simulink model "UAV_6DOF"  (R2024b)
settings: Solver=ode3  StartTime=0.0  StopTime=5.0  FixedStep=0.001  RelTol=1e-3
model workspace (MAT data in the model file):
  Kd_roll = 0.2
  Kd_x = 2
  Kd_y = 1
  Kd_z = 0.3
  Kp_pitch = 0.5
  Kp_roll = 0.5
  Kp_x = 0.9
  Kp_y = -0.9
  Kp_z = -0.9
values from neighbouring files (symbols this model uses):
  mass = 1.5 + rand*0.5    [MonteCarlo.m]
libraries: shared6dof x1
settings Model: Creator=nikhilranjit  LastModifiedBy=nikhilranjit

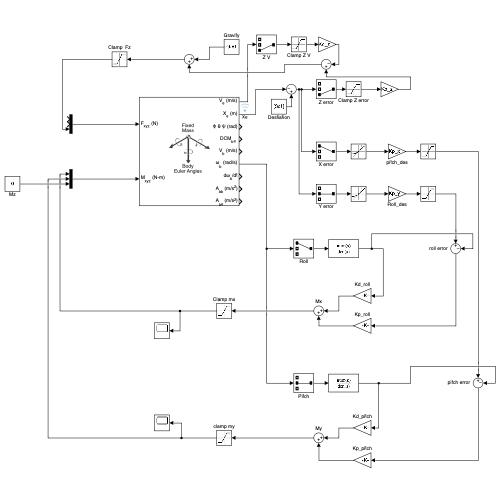
[thumbnail: Simulink's stored preview of the top-level diagram]
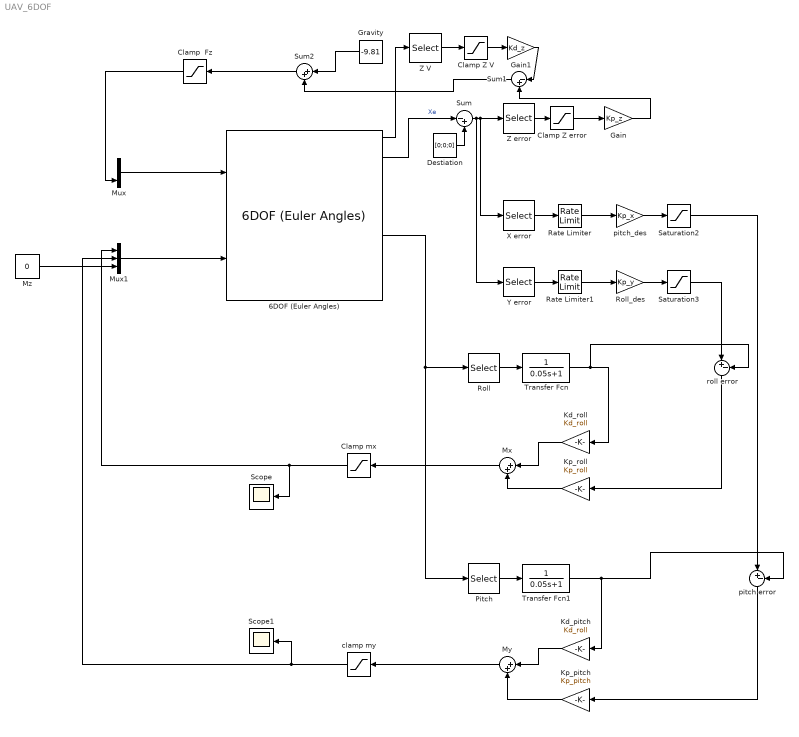
== system UAV_6DOF ==
  6DOF (Euler Angles) : shared6dof/6DOF (Euler Angles)  units=Metric (MKS)  mtype=Fixed  rep=Euler Angles  xme_0=[10 10 0]  Vm_0=[0 0 0]  eul_0=[0 0 0]  pm_0=[0 0 0]  mass_0=1.0  mass_e=0.5  mass_f=2.0  inertia=eye(3)  inertia_e=eye(3)  inertia_f=2*eye(3)  k_quat=1.0  vre_flag=on  abi_flag=on  aMode=0  xme_statename=''  Vm_statename=''  eul_statename=''  quat_statename=''  pm_statename=''  mass_statename=''
  Clamp  Fz : Saturate  UpperLimit=mass*9.81*1.5  LowerLimit=mass*9.81*0.8
  Clamp Z V : Saturate  UpperLimit=5  LowerLimit=-5
  Clamp Z error : Saturate  UpperLimit=5  LowerLimit=-5
  Clamp mx : Saturate  UpperLimit=5  LowerLimit=-5
  Destiation : Constant  Value=[0;0;0]
  Gain : Gain  Gain=Kp_z
  Gain1 : Gain  Gain=Kd_z
  Gravity : Constant  Value=-9.81
  Kd_pitch : Gain  Gain=Kd_roll
  Kd_roll : Gain  Gain=Kd_roll
  Kp_pitch : Gain  Gain=Kp_pitch
  Kp_roll : Gain  Gain=Kp_roll
  Mux : Mux  Inputs=3
  Mux1 : Mux  Inputs=3
  Mx : Sum  Inputs=|++
  My : Sum  Inputs=|++
  Mz : Constant  Value=0
  Pitch : Selector  InputPortWidth=3  IndexOptions=Index vector (dialog)  Indices=2  OutputSizes=1
  Rate Limiter : RateLimiter  SampleTimeMode=inherited
  Rate Limiter1 : RateLimiter  SampleTimeMode=inherited
  Roll : Selector  InputPortWidth=3  IndexOptions=Index vector (dialog)  Indices=1  OutputSizes=1
  Roll_des : Gain  Gain=Kp_y
  Saturation2 : Saturate  UpperLimit=20  LowerLimit=-20
  Saturation3 : Saturate  UpperLimit=20  LowerLimit=-20
  Scope : Scope
  Scope1 : Scope
  Sum : Sum  Inputs=|-+
  Sum1 : Sum  Inputs=|-+
  Sum2 : Sum  Inputs=|++
  Transfer Fcn : TransferFcn  Denominator=[0.05 1]
  Transfer Fcn1 : TransferFcn  Denominator=[0.05 1]
  X error : Selector  InputPortWidth=3  IndexOptions=Index vector (dialog)  Indices=1  OutputSizes=1
  Y error : Selector  InputPortWidth=3  IndexOptions=Index vector (dialog)  Indices=2  OutputSizes=1
  Z V : Selector  InputPortWidth=3  IndexOptions=Index vector (dialog)  Indices=3  OutputSizes=1
  Z error : Selector  InputPortWidth=3  IndexOptions=Index vector (dialog)  Indices=3  OutputSizes=1
  clamp my : Saturate  UpperLimit=5  LowerLimit=-5
  pitch error : Sum  Inputs=|+-
  pitch_des : Gain  Gain=Kp_x
  roll error : Sum  Inputs=|+-
  wires:
  Destiation/1 -> Sum/2
  6DOF (Euler Angles)/2 -> Sum/1  "Xe"
  Sum/1 -> Y error/1, X error/1, Z error/1
  Mux/1 -> 6DOF (Euler Angles)/1
  X error/1 -> Rate Limiter/1
  Y error/1 -> Rate Limiter1/1
  Mux1/1 -> 6DOF (Euler Angles)/2
  Roll_des/1 -> Saturation3/1
  Roll/1 -> Transfer Fcn/1
  roll error/1 -> Kp_roll/1
  Kd_roll/1 -> Mx/1
  pitch_des/1 -> Saturation2/1
  Pitch/1 -> Transfer Fcn1/1
  pitch error/1 -> Kp_pitch/1
  Kd_pitch/1 -> My/1
  Mx/1 -> Clamp mx/1
  My/1 -> clamp my/1
  Mz/1 -> Mux1/3
  Clamp mx/1 -> Scope/1, Mux1/1
  clamp my/1 -> Scope1/1, Mux1/2
  6DOF (Euler Angles)/6 -> Pitch/1, Roll/1
  Kp_pitch/1 -> My/2
  Kp_roll/1 -> Mx/2
  Saturation2/1 -> pitch error/1
  Saturation3/1 -> roll error/1
  Transfer Fcn1/1 -> Kd_pitch/1, pitch error/2
  Transfer Fcn/1 -> Kd_roll/1, roll error/2
  Rate Limiter/1 -> pitch_des/1
  Rate Limiter1/1 -> Roll_des/1
  6DOF (Euler Angles)/1 -> Z V/1
  Z V/1 -> Clamp Z V/1
  Z error/1 -> Clamp Z error/1
  Clamp Z error/1 -> Gain/1
  Gain1/1 -> Sum1/1
  Gain/1 -> Sum1/2
  Sum1/1 -> Sum2/2
  Sum2/1 -> Clamp  Fz/1
  Clamp Z V/1 -> Gain1/1
  Clamp  Fz/1 -> Mux/3
  Gravity/1 -> Sum2/1
